simulink model "BLDC_Control_Logic"  (R2017b)
settings: Solver=FixedStepDiscrete  StartTime=0.0  StopTime=10  RelTol=1e-3
libraries: pePwmGenerator x1, simulink x1
settings Model: SimulationMode=accelerator  Creator=proso  LastModifiedBy=proso
settings DataIOCC: SaveOutput=off  SaveTime=off
settings OptimizationCC: DefaultParameterBehavior=Inlined  PassReuseOutputArgsAs=Individual arguments
settings DebuggingCC: ParameterTunabilityLossMsg=error
settings SFSimCC: MATLABDynamicMemAlloc=off
settings RTWCC: SystemTargetFile=ert.tlc  TemplateMakefile=ert_default_tmf  GenerateReport=on  IncludeHyperlinkInReport=on  LaunchReport=on  GenerateTraceInfo=on  GenerateTraceReport=on  GenerateTraceReportSl=on  GenerateTraceReportSf=on  GenerateTraceReportEml=on
settings CodeAppCC: ForceParamTrailComments=on  IgnoreCustomStorageClasses=off  OperatorAnnotations=on  SimulinkDataObjDesc=on  SFDataObjDesc=on  InsertBlockDesc=on
settings ERTTargetCC: TargetLangStandard=C99 (ISO)  GenerateSampleERTMain=on  InlinedParameterPlacement=NonHierarchical  ERTCustomFileTemplate=example_file_process.tlc

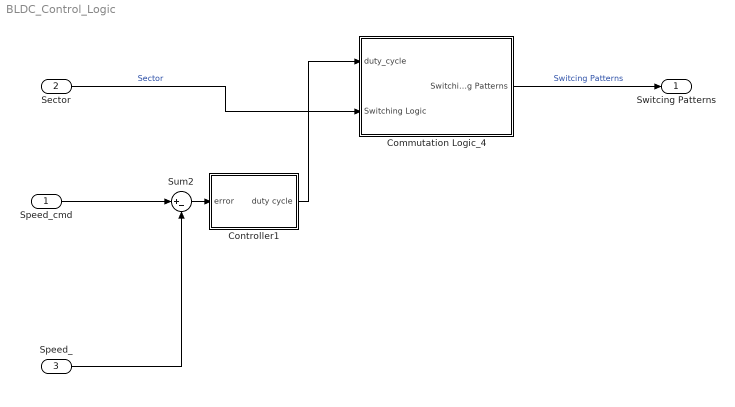
== system BLDC_Control_Logic ==
  Speed_cmd : Inport  OutDataTypeStr=double  PortDimensions=1  SampleTime=[1.0000000000000001e-05,0]
  Sector : Inport  Port=2  OutDataTypeStr=double  PortDimensions=6  SampleTime=[1.0000000000000001e-05,0]
  Speed_ : Inport  Port=3  OutDataTypeStr=double  PortDimensions=1  SampleTime=[1.0000000000000001e-05,0]
  Commutation Logic_4 : Subsystem
  Controller1 : Subsystem
  Sum2 : Sum  Inputs=|+-
  Switcing Patterns : Outport  OutDataTypeStr=double  PortDimensions=6  SampleTime=[1.0000000000000001e-05,0]
  wires:
  Speed_/1 -> Sum2/2
  Commutation Logic_4/1(Switching Patterns) -> Switcing Patterns/1  "Switcing Patterns"
  Controller1/1(duty cycle) -> Commutation Logic_4/1(duty_cycle)
  Sector/1 -> Commutation Logic_4/2(Switching Logic)  "Sector"
  Sum2/1 -> Controller1/1(error)
  Speed_cmd/1 -> Sum2/1

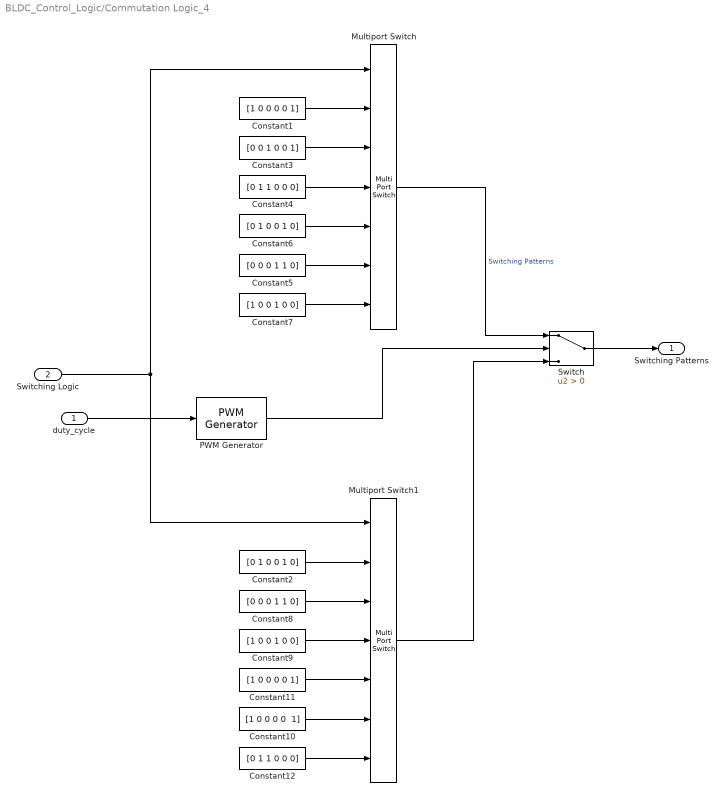
== system BLDC_Control_Logic/Commutation Logic_4 ==
  duty_cycle : Inport
  Switching Logic : Inport  Port=2
  Constant1 : Constant  Value=[1 0 0 0 0 1]
  Constant10 : Constant  Value="[1 0 0 0 0  1]"
  Constant11 : Constant  Value=[1 0 0 0 0 1]
  Constant12 : Constant  Value=[0 1 1 0 0 0]
  Constant2 : Constant  Value=[0 1 0 0 1 0]
  Constant3 : Constant  Value=[0 0 1 0 0 1]
  Constant4 : Constant  Value=[0 1 1 0 0 0]
  Constant5 : Constant  Value=[0 0 0 1 1 0]
  Constant6 : Constant  Value=[0 1 0 0 1 0]
  Constant7 : Constant  Value=[1 0 0 1 0 0]
  Constant8 : Constant  Value=[0 0 0 1 1 0]
  Constant9 : Constant  Value=[1 0 0 1 0 0]
  Multiport Switch : MultiPortSwitch  DataPortOrder=Zero-based contiguous  Inputs=6
  Multiport Switch1 : MultiPortSwitch  DataPortOrder=Zero-based contiguous  Inputs=6
  PWM Generator : pePwmGenerator/PWM Generator  CarrCount=Up  Tper=0.001  Ts=5e-5
  Switch : Switch  Criteria=u2 > Threshold
  Switching Patterns : Outport
  wires:
  Multiport Switch1/1 -> Switch/3
  Constant11/1 -> Multiport Switch1/5
  Constant10/1 -> Multiport Switch1/6
  Constant2/1 -> Multiport Switch1/2
  Constant8/1 -> Multiport Switch1/3
  Constant9/1 -> Multiport Switch1/4
  Constant12/1 -> Multiport Switch1/7
  Switch/1 -> Switching Patterns/1
  Multiport Switch/1 -> Switch/1  "Switching Patterns"
  PWM Generator/1 -> Switch/2
  duty_cycle/1 -> PWM Generator/1
  Constant5/1 -> Multiport Switch/6
  Constant6/1 -> Multiport Switch/5
  Constant3/1 -> Multiport Switch/3
  Constant7/1 -> Multiport Switch/7
  Constant1/1 -> Multiport Switch/2
  Constant4/1 -> Multiport Switch/4
  Switching Logic/1 -> Multiport Switch/1, Multiport Switch1/1

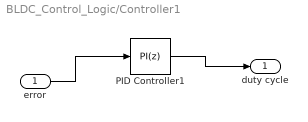
== system BLDC_Control_Logic/Controller1 ==
  error : Inport
  PID Controller1 : simulink/Continuous/PID Controller  Controller=PI  TimeDomain=Discrete-time  SampleTime=-1  IntegratorMethod=Forward Euler  FilterMethod=Forward Euler  Form=Parallel  UseFilter=on  ControllerParametersSource=internal  P=0.01  I=5  D=0  N=100  InitialConditionSource=internal  InitialConditionForIntegrator=0  InitialConditionForFilter=0  ExternalReset=none  LimitOutput=off  UpperSaturationLimit=inf  LowerSaturationLimit=-inf  LinearizeAsGain=on  AntiWindupMode=none  Kb=1  TrackingMode=off  Kt=1  PParamMin=[]  PParamMax=[]  IParamMin=[]  IParamMax=[]  DParamMin=[]  DParamMax=[]  NParamMin=[]  NParamMax=[]  KbParamMin=[]  KbParamMax=[]  KtParamMin=[]  KtParamMax=[]  POutMin=[]  POutMax=[]  IOutMin=[]  IOutMax=[]  DOutMin=[]  DOutMax=[]  NOutMin=[]  NOutMax=[]  KbOutMin=[]  KbOutMax=[]  KtOutMin=[]  KtOutMax=[]  IntegratorOutMin=[]  IntegratorOutMax=[]  FilterOutMin=[]  FilterOutMax=[]  SumOutMin=[]  SumOutMax=[]  SumI1OutMin=[]  SumI1OutMax=[]  SumI2OutMin=[]  SumI2OutMax=[]  SumI3OutMin=[]  SumI3OutMax=[]  SumDOutMin=[]  SumDOutMax=[]  SaturationOutMin=[]  SaturationOutMax=[]  IntegratorContinuousStateAttributes=''  IntegratorStateMustResolveToSignalObject=off  IntegratorRTWStateStorageClass=Auto  FilterContinuousStateAttributes=''  FilterStateMustResolveToSignalObject=off  FilterRTWStateStorageClass=Auto  DifferentiatorICPrevScaledInput=0  DifferentiatorOutMin=[]  DifferentiatorOutMax=[]  InitialConditionSetting=State (most efficient)  FilterDiffOutCoefMin=[]  FilterDiffOutCoefMax=[]  SumDenOutMin=[]  SumDenOutMax=[]  SumNumOutMin=[]  SumNumOutMax=[]  ReciprocalOutMin=[]  ReciprocalOutMax=[]  DivideOutMin=[]  DivideOutMax=[]  TunerSelectOption=Transfer Function Based (PID Tuner App)
  duty cycle : Outport
  wires:
  error/1 -> PID Controller1/1
  PID Controller1/1 -> duty cycle/1
